simulink model "Motor_Fault_healthy"  (R2025b)
settings: Solver=ode4  StartTime=0.0  StopTime=10  FixedStep=0.01  RelTol=1e-3
settings Model: Creator=anifa  LastModifiedBy=anifa

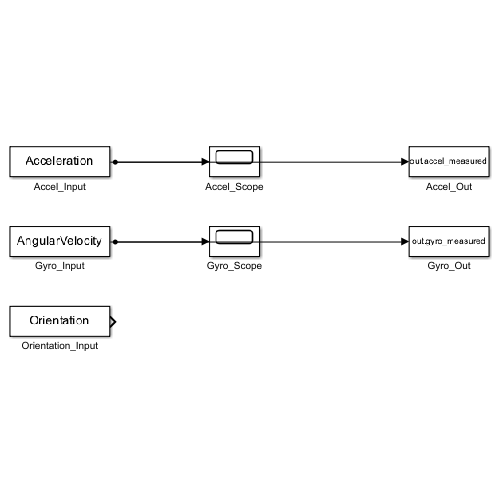
[thumbnail: Simulink's stored preview of the top-level diagram]
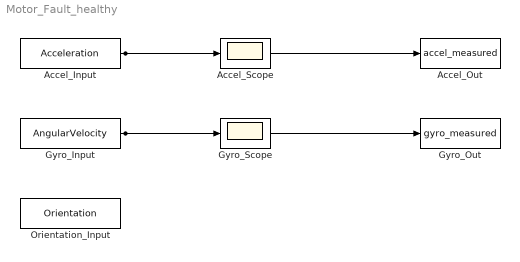
== system Motor_Fault_healthy ==
  Accel_Input : FromWorkspace  VariableName=Acceleration
  Accel_Out : ToWorkspace  VariableName=accel_measured  SaveFormat=Timeseries  SampleTime=-1
  Accel_Scope : Scope
  Gyro_Input : FromWorkspace  VariableName=AngularVelocity
  Gyro_Out : ToWorkspace  VariableName=gyro_measured  SaveFormat=Timeseries  SampleTime=-1
  Gyro_Scope : Scope
  Orientation_Input : FromWorkspace  VariableName=Orientation
  wires:
  Accel_Input/1 -> Accel_Scope/1, Accel_Out/1
  Gyro_Input/1 -> Gyro_Scope/1, Gyro_Out/1
